simulink model "Laboratorio_6_SC2_Simulink"  (R2019a)
settings: Solver=VariableStepAuto  StartTime=0.0  StopTime=4  RelTol=1e-3
values from neighbouring files (symbols this model uses):
  A_cl = A - (B * K_pp)    [Laboratorio_6_SC2.m]
  A_cl_s2 = A - (B * K_pp_s2)    [Laboratorio_6_SC2.m]
  B = [1/(r1*c1);0;0]    [Laboratorio_6_SC2.m]
  C = [-0 1 0]    [Laboratorio_6_SC2.m]
  D = 0    [Laboratorio_6_SC2.m]
  K_pp = place(A, B, p)    [Laboratorio_6_SC2.m]
  K_pp_s2 = place(A, B, p_s2)    [Laboratorio_6_SC2.m]
  Nbar = rscale(sys, K_pp)    [Laboratorio_6_SC2.m]
  Nbar_2 = rscale(sys, K_pp_s2)    [Laboratorio_6_SC2.m]
  r1 = 1e3    (= 1000)    [Laboratorio_6_SC2.m]
  r2 = 10e3    (= 10000)    [Laboratorio_6_SC2.m]
  r3 = r2    (= 10000)    [Laboratorio_6_SC2.m]
libraries: fl_lib x24, nesl_utility x14, ee_lib x6
settings Model: Creator=Hector  LastModifiedBy=Hector

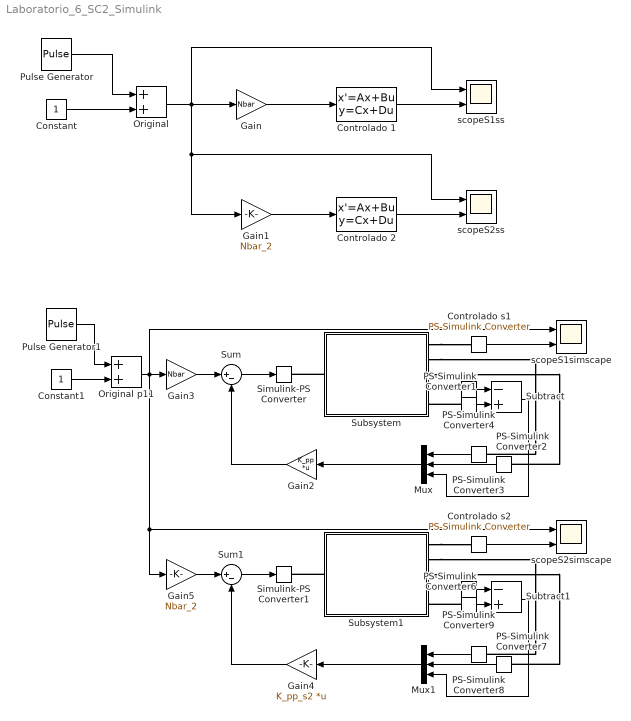
== system Laboratorio_6_SC2_Simulink ==
  Constant : Constant
  Constant1 : Constant
  Controlado 1 : StateSpace  A=A_cl  B=B  C=C  D=D  InitialCondition=0
  Controlado 2 : StateSpace  A=A_cl_s2  B=B  C=C  D=D  InitialCondition=0
  Controlado s1 : nesl_utility/PS-Simulink Converter  PhysicalDomain=network_engine_domain  SubClassName=ps_output  LeftPortType=input  RightPortType=output  PseudoPeriodic=off  Frequencies=[]  Unit=1  AffineConversion=off
  "Controlado s2 " : nesl_utility/PS-Simulink Converter  PhysicalDomain=network_engine_domain  SubClassName=ps_output  LeftPortType=input  RightPortType=output  PseudoPeriodic=off  Frequencies=[]  Unit=1  AffineConversion=off
  Gain : Gain  Gain=Nbar
  Gain1 : Gain  Gain=Nbar_2
  Gain2 : Gain  Gain=K_pp  Multiplication=Matrix(K*u) (u vector)
  Gain3 : Gain  Gain=Nbar
  Gain4 : Gain  Gain=K_pp_s2  Multiplication=Matrix(K*u) (u vector)
  Gain5 : Gain  Gain=Nbar_2
  Mux : Mux  Inputs=3
  Mux1 : Mux  Inputs=3
  Original : Sum
  Original p11 : Sum
  PS-Simulink Converter{1..4,6..9} (8 alike) : nesl_utility/PS-Simulink Converter  PhysicalDomain=network_engine_domain  SubClassName=ps_output  LeftPortType=input  RightPortType=output  PseudoPeriodic=off  Frequencies=[]  Unit=1  AffineConversion=off
  Pulse Generator : DiscretePulseGenerator  PulseType=Time based  Period=1/0.5  PulseWidth=50
  Pulse Generator1 : DiscretePulseGenerator  PulseType=Time based  Period=1/0.5  PulseWidth=50
  Simulink-PS Converter : nesl_utility/Simulink-PS Converter  PhysicalDomain=network_engine_domain  SubClassName=ps_input  LeftPortType=input  RightPortType=output  PseudoPeriodic=off  Frequencies=[]  NoiseDistribution=none  NoiseParameters=[]  Unit=1  AffineConversion=off  FilteringAndDerivatives=provide  SimscapeFilterOrder=1  InputFilterTimeConstant=0.001  UdotUserProvided=0
  Simulink-PS Converter1 : nesl_utility/Simulink-PS Converter  PhysicalDomain=network_engine_domain  SubClassName=ps_input  LeftPortType=input  RightPortType=output  PseudoPeriodic=off  Frequencies=[]  NoiseDistribution=none  NoiseParameters=[]  Unit=1  AffineConversion=off  FilteringAndDerivatives=provide  SimscapeFilterOrder=1  InputFilterTimeConstant=0.001  UdotUserProvided=0
  Subsystem : Subsystem
  Subsystem1 : Subsystem
  Subtract : Sum  Inputs=-+
  Subtract1 : Sum  Inputs=-+
  Sum : Sum  Inputs=|+-
  Sum1 : Sum  Inputs=|+-
  scopeS1simscape : Scope  NumInputPorts=2
  scopeS1ss : Scope  NumInputPorts=2
  scopeS2simscape : Scope  NumInputPorts=2
  scopeS2ss : Scope  NumInputPorts=2
  wires:
  Pulse Generator/1 -> Original/1
  Constant/1 -> Original/2
  Gain/1 -> Controlado 1/1
  Controlado 1/1 -> scopeS1ss/2
  Controlado s1/1 -> scopeS1simscape/2
  Original/1 -> scopeS2ss/1, Gain1/1, scopeS1ss/1, Gain/1
  Controlado 2/1 -> scopeS2ss/2
  Gain1/1 -> Controlado 2/1
  Constant1/1 -> Original p11/2
  Pulse Generator1/1 -> Original p11/1
  Gain2/1 -> Sum/2
  Sum/1 -> Simulink-PS Converter/1
  Gain3/1 -> Sum/1
  PS-Simulink Converter2/1 -> Mux/2
  PS-Simulink Converter3/1 -> Mux/1
  Mux/1 -> Gain2/1
  PS-Simulink Converter4/1 -> Subtract/1
  PS-Simulink Converter1/1 -> Subtract/2
  Subtract/1 -> Mux/3
  PS-Simulink Converter7/1 -> Mux1/2
  Sum1/1 -> Simulink-PS Converter1/1
  "Controlado s2 "/1 -> scopeS2simscape/2
  PS-Simulink Converter6/1 -> Subtract1/2
  PS-Simulink Converter9/1 -> Subtract1/1
  Gain4/1 -> Sum1/2
  Mux1/1 -> Gain4/1
  Subtract1/1 -> Mux1/3
  Gain5/1 -> Sum1/1
  PS-Simulink Converter8/1 -> Mux1/1
  Original p11/1 -> Gain3/1, Gain5/1, scopeS2simscape/1, scopeS1simscape/1
  connections:
  Subsystem/RConn1 -- Controlado s1/LConn1
  Subsystem/LConn1 -- Simulink-PS Converter/RConn1
  Subsystem/RConn2 -- PS-Simulink Converter3/LConn1
  Subsystem/RConn3 -- PS-Simulink Converter2/LConn1
  PS-Simulink Converter1/LConn1 -- Subsystem/RConn5
  PS-Simulink Converter4/LConn1 -- Subsystem/RConn4
  PS-Simulink Converter6/LConn1 -- Subsystem1/RConn5
  Subsystem1/RConn2 -- PS-Simulink Converter8/LConn1
  PS-Simulink Converter9/LConn1 -- Subsystem1/RConn4
  Subsystem1/LConn1 -- Simulink-PS Converter1/RConn1
  Subsystem1/RConn1 -- "Controlado s2 "/LConn1
  Subsystem1/RConn3 -- PS-Simulink Converter7/LConn1

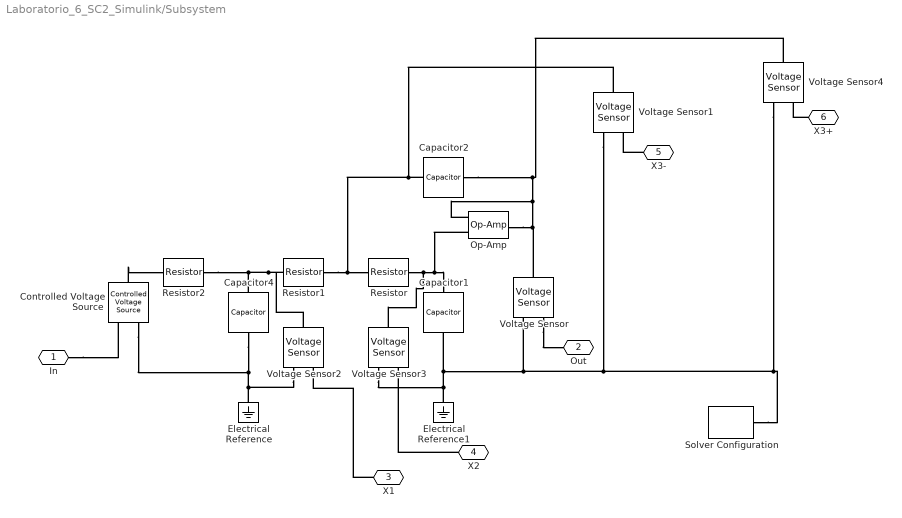
== system Laboratorio_6_SC2_Simulink/Subsystem ==
  Capacitor1 : fl_lib/Electrical/Electrical Elements/Capacitor  c=c2 F  r=0 Ohm  g=0 1/Ohm  i_specify=off  i_priority=None  i=0 A  i_nominal_specify=off  i_nominal_unit=A  i_nominal_value=1  v_specify=off  v_priority=None  v=0 V  v_nominal_specify=off  v_nominal_unit=V  v_nominal_value=1  vc_specify=off  vc_priority=High  vc=0 V  vc_nominal_specify=off  vc_nominal_unit=V  vc_nominal_value=1
  Capacitor2 : fl_lib/Electrical/Electrical Elements/Capacitor  c=c3 F  r=0 Ohm  g=0 1/Ohm  i_specify=off  i_priority=None  i=0 A  i_nominal_specify=off  i_nominal_unit=A  i_nominal_value=1  v_specify=off  v_priority=None  v=0 V  v_nominal_specify=off  v_nominal_unit=V  v_nominal_value=1  vc_specify=off  vc_priority=High  vc=0 V  vc_nominal_specify=off  vc_nominal_unit=V  vc_nominal_value=1
  Capacitor4 : fl_lib/Electrical/Electrical Elements/Capacitor  c=c1 F  r=0 Ohm  g=0 1/Ohm  i_specify=off  i_priority=None  i=0 A  i_nominal_specify=off  i_nominal_unit=A  i_nominal_value=1  v_specify=off  v_priority=None  v=0 V  v_nominal_specify=off  v_nominal_unit=V  v_nominal_value=1  vc_specify=off  vc_priority=High  vc=0 V  vc_nominal_specify=off  vc_nominal_unit=V  vc_nominal_value=1
  Controlled Voltage Source : fl_lib/Electrical/Electrical Sources/Controlled Voltage Source
  Electrical Reference : fl_lib/Electrical/Electrical Elements/Electrical Reference
  Electrical Reference1 : fl_lib/Electrical/Electrical Elements/Electrical Reference
  Op-Amp : fl_lib/Electrical/Electrical Elements/Op-Amp  outI_specify=off  outI_priority=None  outI=0 A  outI_nominal_specify=off  outI_nominal_unit=A  outI_nominal_value=1
  Resistor : ee_lib/Passive/Resistor  R=r3 Ohm  R_tol=5  enable_R_tol=0  tol_distribution=1  nSigma=4  enable_operating_limits=0  operating_limit_action=2  max_working_voltage=100 V  power_rating=1 W  enable_faults=0  fault_action=1  R_faulted=inf Ohm  enable_temporal_fault=0  t_fault=1 s  enable_behavioral_fault=0  max_permissible_current=1 A  t_fail_on_current=1 s  noise_mode=0  sample_time=1e-3 s  repeatability=1  auto_seed=3922919431  user_seed=0  Tdevice=25 degC  alpha=3.93e-3 1/K  Tmeas=25 degC  thermal_mass=100 J/K  power_derating_T1=70 degC  power_derating_T2=155 degC  operating_temperature_range_vec=[-50, 150] degC  temperature_specify=off  temperature_priority=High  temperature=298.15 K  temperature_nominal_specify=off  temperature_nominal_unit=K  temperature_nominal_value=1
      settings: SourceProductName=Simscape Electrical
  Resistor1 : ee_lib/Passive/Resistor  R=r2 Ohm  R_tol=5  enable_R_tol=0  tol_distribution=1  nSigma=4  enable_operating_limits=0  operating_limit_action=2  max_working_voltage=100 V  power_rating=1 W  enable_faults=0  fault_action=1  R_faulted=inf Ohm  enable_temporal_fault=0  t_fault=1 s  enable_behavioral_fault=0  max_permissible_current=1 A  t_fail_on_current=1 s  noise_mode=0  sample_time=1e-3 s  repeatability=1  auto_seed=2715962282  user_seed=0  Tdevice=25 degC  alpha=3.93e-3 1/K  Tmeas=25 degC  thermal_mass=100 J/K  power_derating_T1=70 degC  power_derating_T2=155 degC  operating_temperature_range_vec=[-50, 150] degC  temperature_specify=off  temperature_priority=High  temperature=298.15 K  temperature_nominal_specify=off  temperature_nominal_unit=K  temperature_nominal_value=1
      settings: SourceProductName=Simscape Electrical
  Resistor2 : ee_lib/Passive/Resistor  R=r1 Ohm  R_tol=5  enable_R_tol=0  tol_distribution=1  nSigma=4  enable_operating_limits=0  operating_limit_action=2  max_working_voltage=100 V  power_rating=1 W  enable_faults=0  fault_action=1  R_faulted=inf Ohm  enable_temporal_fault=0  t_fault=1 s  enable_behavioral_fault=0  max_permissible_current=1 A  t_fail_on_current=1 s  noise_mode=0  sample_time=1e-3 s  repeatability=1  auto_seed=418932850  user_seed=0  Tdevice=25 degC  alpha=3.93e-3 1/K  Tmeas=25 degC  thermal_mass=100 J/K  power_derating_T1=70 degC  power_derating_T2=155 degC  operating_temperature_range_vec=[-50, 150] degC  temperature_specify=off  temperature_priority=High  temperature=298.15 K  temperature_nominal_specify=off  temperature_nominal_unit=K  temperature_nominal_value=1
      settings: SourceProductName=Simscape Electrical
  Solver Configuration : nesl_utility/Solver Configuration  PhysicalDomain=network_engine_domain  SubClassName=solver  LeftPortType=input  RightPortType=generic  Tones=[]  Harmonics=[]  SimulateNoise=off  Profile=off  UseLocalSampling=off  EnableSwitchedLinearOptims=on  FrequencyDomain=off  UseCCode=off  RelTol=0.001  AbsTol=1e-06  MinStep=1e-09  ToWorkspace=off  RevertToSquareIcSolve=off  NumHomotopyIterations=100  PhasorMode=off  PhasorModeNumHarmonics=1  DoDC=off  ResidualTolerance=1e-09  UseLocalSolver=off  LocalSolverChoice=NE_BACKWARD_EULER_ADVANCER  LocalSolverSampleTime=0.001  DoFixedCost=off  MaxNonlinIter=3  MaxModeIter=2  LinearAlgebra=auto  EquationFormulation=NE_TIME_EF  DelaysMemoryBudget=1024  AutomaticFiltering=on  FilteringTimeConstant=0.001  PartitionStorageMethod=AS_NEEDED  PartitionMemoryBudget=1024  PartitionMethod=FAST
  Voltage Sensor{,1..4} (5 alike) : fl_lib/Electrical/Electrical Sensors/Voltage Sensor
  In : PMIOPort  Side=Left
  "Out " : PMIOPort  Port=2  Side=Right
  X1 : PMIOPort  Port=3  Side=Right
  X2 : PMIOPort  Port=4  Side=Right
  X3- : PMIOPort  Port=5  Side=Right
  "X3+ " : PMIOPort  Port=6  Side=Right
  connections:
  Capacitor1/RConn1 -- Voltage Sensor3/RConn2 -- Electrical Reference1/LConn1 -- Voltage Sensor4/RConn2 -- Solver Configuration/RConn1 -- Voltage Sensor1/RConn2 -- Voltage Sensor/RConn2
  Capacitor4/LConn1 -- Resistor2/RConn1 -- Voltage Sensor2/LConn1 -- Resistor1/LConn1
  Resistor1/RConn1 -- Capacitor2/LConn1 -- Voltage Sensor1/LConn1 -- Resistor/LConn1
  Controlled Voltage Source/RConn2 -- Capacitor4/RConn1 -- Electrical Reference/LConn1 -- Voltage Sensor2/RConn2
  Resistor/RConn1 -- Voltage Sensor3/LConn1 -- Op-Amp/LConn1 -- Capacitor1/LConn1
  Op-Amp/RConn1 -- Capacitor2/RConn1 -- Voltage Sensor4/LConn1 -- Op-Amp/LConn2 -- Voltage Sensor/LConn1
  "X3+ "/RConn1 -- Voltage Sensor4/RConn1
  Controlled Voltage Source/LConn1 -- Resistor2/LConn1
  In/RConn1 -- Controlled Voltage Source/RConn1
  X2/RConn1 -- Voltage Sensor3/RConn1
  X1/RConn1 -- Voltage Sensor2/RConn1
  Voltage Sensor/RConn1 -- "Out "/RConn1
  X3-/RConn1 -- Voltage Sensor1/RConn1

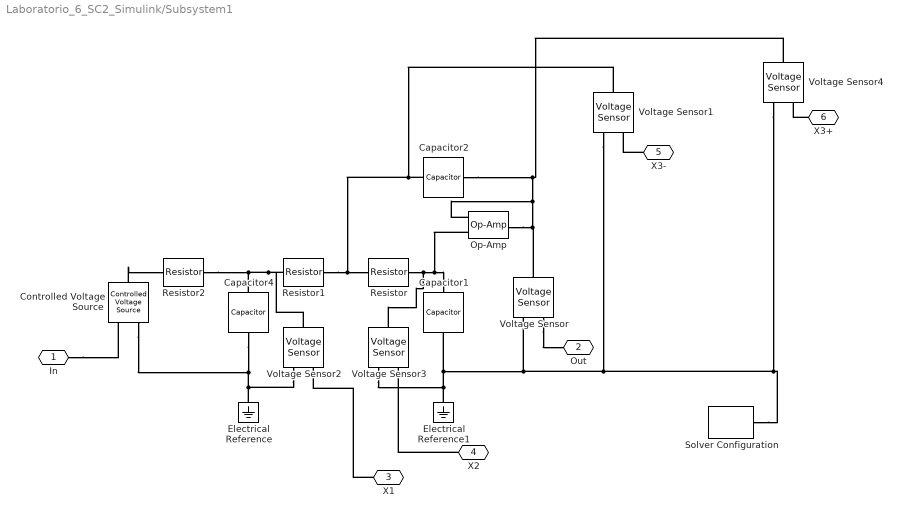
== system Laboratorio_6_SC2_Simulink/Subsystem1 ==
  Capacitor1 : fl_lib/Electrical/Electrical Elements/Capacitor  c=c2 F  r=0 Ohm  g=0 1/Ohm  i_specify=off  i_priority=None  i=0 A  i_nominal_specify=off  i_nominal_unit=A  i_nominal_value=1  v_specify=off  v_priority=None  v=0 V  v_nominal_specify=off  v_nominal_unit=V  v_nominal_value=1  vc_specify=off  vc_priority=High  vc=0 V  vc_nominal_specify=off  vc_nominal_unit=V  vc_nominal_value=1
  Capacitor2 : fl_lib/Electrical/Electrical Elements/Capacitor  c=c3 F  r=0 Ohm  g=0 1/Ohm  i_specify=off  i_priority=None  i=0 A  i_nominal_specify=off  i_nominal_unit=A  i_nominal_value=1  v_specify=off  v_priority=None  v=0 V  v_nominal_specify=off  v_nominal_unit=V  v_nominal_value=1  vc_specify=off  vc_priority=High  vc=0 V  vc_nominal_specify=off  vc_nominal_unit=V  vc_nominal_value=1
  Capacitor4 : fl_lib/Electrical/Electrical Elements/Capacitor  c=c1 F  r=0 Ohm  g=0 1/Ohm  i_specify=off  i_priority=None  i=0 A  i_nominal_specify=off  i_nominal_unit=A  i_nominal_value=1  v_specify=off  v_priority=None  v=0 V  v_nominal_specify=off  v_nominal_unit=V  v_nominal_value=1  vc_specify=off  vc_priority=High  vc=0 V  vc_nominal_specify=off  vc_nominal_unit=V  vc_nominal_value=1
  Controlled Voltage Source : fl_lib/Electrical/Electrical Sources/Controlled Voltage Source
  Electrical Reference : fl_lib/Electrical/Electrical Elements/Electrical Reference
  Electrical Reference1 : fl_lib/Electrical/Electrical Elements/Electrical Reference
  Op-Amp : fl_lib/Electrical/Electrical Elements/Op-Amp  outI_specify=off  outI_priority=None  outI=0 A  outI_nominal_specify=off  outI_nominal_unit=A  outI_nominal_value=1
  Resistor : ee_lib/Passive/Resistor  R=r3 Ohm  R_tol=5  enable_R_tol=0  tol_distribution=1  nSigma=4  enable_operating_limits=0  operating_limit_action=2  max_working_voltage=100 V  power_rating=1 W  enable_faults=0  fault_action=1  R_faulted=inf Ohm  enable_temporal_fault=0  t_fault=1 s  enable_behavioral_fault=0  max_permissible_current=1 A  t_fail_on_current=1 s  noise_mode=0  sample_time=1e-3 s  repeatability=1  auto_seed=3499211588  user_seed=0  Tdevice=25 degC  alpha=3.93e-3 1/K  Tmeas=25 degC  thermal_mass=100 J/K  power_derating_T1=70 degC  power_derating_T2=155 degC  operating_temperature_range_vec=[-50, 150] degC  temperature_specify=off  temperature_priority=High  temperature=298.15 K  temperature_nominal_specify=off  temperature_nominal_unit=K  temperature_nominal_value=1
      settings: SourceProductName=Simscape Electrical
  Resistor1 : ee_lib/Passive/Resistor  R=r2 Ohm  R_tol=5  enable_R_tol=0  tol_distribution=1  nSigma=4  enable_operating_limits=0  operating_limit_action=2  max_working_voltage=100 V  power_rating=1 W  enable_faults=0  fault_action=1  R_faulted=inf Ohm  enable_temporal_fault=0  t_fault=1 s  enable_behavioral_fault=0  max_permissible_current=1 A  t_fail_on_current=1 s  noise_mode=0  sample_time=1e-3 s  repeatability=1  auto_seed=3890346746  user_seed=0  Tdevice=25 degC  alpha=3.93e-3 1/K  Tmeas=25 degC  thermal_mass=100 J/K  power_derating_T1=70 degC  power_derating_T2=155 degC  operating_temperature_range_vec=[-50, 150] degC  temperature_specify=off  temperature_priority=High  temperature=298.15 K  temperature_nominal_specify=off  temperature_nominal_unit=K  temperature_nominal_value=1
      settings: SourceProductName=Simscape Electrical
  Resistor2 : ee_lib/Passive/Resistor  R=r1 Ohm  R_tol=5  enable_R_tol=0  tol_distribution=1  nSigma=4  enable_operating_limits=0  operating_limit_action=2  max_working_voltage=100 V  power_rating=1 W  enable_faults=0  fault_action=1  R_faulted=inf Ohm  enable_temporal_fault=0  t_fault=1 s  enable_behavioral_fault=0  max_permissible_current=1 A  t_fail_on_current=1 s  noise_mode=0  sample_time=1e-3 s  repeatability=1  auto_seed=545404223  user_seed=0  Tdevice=25 degC  alpha=3.93e-3 1/K  Tmeas=25 degC  thermal_mass=100 J/K  power_derating_T1=70 degC  power_derating_T2=155 degC  operating_temperature_range_vec=[-50, 150] degC  temperature_specify=off  temperature_priority=High  temperature=298.15 K  temperature_nominal_specify=off  temperature_nominal_unit=K  temperature_nominal_value=1
      settings: SourceProductName=Simscape Electrical
  Solver Configuration : nesl_utility/Solver Configuration  PhysicalDomain=network_engine_domain  SubClassName=solver  LeftPortType=input  RightPortType=generic  Tones=[]  Harmonics=[]  SimulateNoise=off  Profile=off  UseLocalSampling=off  EnableSwitchedLinearOptims=on  FrequencyDomain=off  UseCCode=off  RelTol=0.001  AbsTol=1e-06  MinStep=1e-09  ToWorkspace=off  RevertToSquareIcSolve=off  NumHomotopyIterations=100  PhasorMode=off  PhasorModeNumHarmonics=1  DoDC=off  ResidualTolerance=1e-09  UseLocalSolver=off  LocalSolverChoice=NE_BACKWARD_EULER_ADVANCER  LocalSolverSampleTime=0.001  DoFixedCost=off  MaxNonlinIter=3  MaxModeIter=2  LinearAlgebra=auto  EquationFormulation=NE_TIME_EF  DelaysMemoryBudget=1024  AutomaticFiltering=on  FilteringTimeConstant=0.001  PartitionStorageMethod=AS_NEEDED  PartitionMemoryBudget=1024  PartitionMethod=FAST
  Voltage Sensor{,1..4} (5 alike) : fl_lib/Electrical/Electrical Sensors/Voltage Sensor
  In : PMIOPort  Side=Left
  "Out " : PMIOPort  Port=2  Side=Right
  X1 : PMIOPort  Port=3  Side=Right
  X2 : PMIOPort  Port=4  Side=Right
  X3- : PMIOPort  Port=5  Side=Right
  "X3+ " : PMIOPort  Port=6  Side=Right
  connections:
  Capacitor1/RConn1 -- Voltage Sensor3/RConn2 -- Electrical Reference1/LConn1 -- Voltage Sensor4/RConn2 -- Solver Configuration/RConn1 -- Voltage Sensor1/RConn2 -- Voltage Sensor/RConn2
  Capacitor4/LConn1 -- Resistor2/RConn1 -- Voltage Sensor2/LConn1 -- Resistor1/LConn1
  Resistor1/RConn1 -- Capacitor2/LConn1 -- Voltage Sensor1/LConn1 -- Resistor/LConn1
  Controlled Voltage Source/RConn2 -- Capacitor4/RConn1 -- Electrical Reference/LConn1 -- Voltage Sensor2/RConn2
  Resistor/RConn1 -- Voltage Sensor3/LConn1 -- Op-Amp/LConn1 -- Capacitor1/LConn1
  Op-Amp/RConn1 -- Capacitor2/RConn1 -- Voltage Sensor4/LConn1 -- Op-Amp/LConn2 -- Voltage Sensor/LConn1
  "X3+ "/RConn1 -- Voltage Sensor4/RConn1
  Controlled Voltage Source/LConn1 -- Resistor2/LConn1
  In/RConn1 -- Controlled Voltage Source/RConn1
  X2/RConn1 -- Voltage Sensor3/RConn1
  X1/RConn1 -- Voltage Sensor2/RConn1
  Voltage Sensor/RConn1 -- "Out "/RConn1
  X3-/RConn1 -- Voltage Sensor1/RConn1
